simulink model "BD_CONV2"  (Simulink 4.1.1)
settings: Solver=ode1  SolverMode=SingleTasking  StartTime=0.0  StopTime=max(cyc_mph(:,1))  FixedStep=1  MaxStep=1  RelTol=1e-3  AbsTol=1e-3
undefined symbols (not defined in the file): cyc_mph, ess_on, ex_calc, fc_ct_trq, fc_emis, fc_inertia, fc_map_spd, fc_max_trq, fc_spd_scale, fc_trq_scale, fd_inertia, fd_loss, fd_ratio, gb_dnshift_load, gb_dnshift_spd, gb_gears_num, gb_inertia, gb_num_init, gb_ratio, gb_shift_delay, gb_spd_scale, gb_trq_scale, gb_upshift_load, gb_upshift_spd, logFlag, tx_eff_map, tx_map_spd, tx_map_trq, vc_clutch_bool, vc_idle_bool, vc_idle_spd, vc_key_on, vc_launch_spd, veh_air_density, veh_CD, veh_FA, veh_gravity, veh_mass, wh_axle_loss_mass, wh_axle_loss_trq, wh_front_active_bool, wh_inertia, wh_max_front_brake_force, wh_max_rear_brake_force, wh_radius, wh_rear_active_bool, wh_slip, wh_slip_force_coeff
libraries: lib_wheel2 x12, lib_drive_cycle2 x2, lib_accessory2 x2, lib_etc x2, lib_interactive x1, lib_exhaust x1, lib_fuel_converter3 x1, lib_help x1
(part 8 of 11)

== system BD_CONV2/<cs> control strategy/Clutch Control/Clutch Control/clutch control ==
  shifting : Inport  Port=1  LatchInput=off
  gb_trq_in_r : Inport  Port=2  LatchInput=off
  gb_spd_in_r : Inport  Port=3  LatchInput=off
  Block NOTES : Subsystem
      settings: RTWFcnNameOpts=Auto  RTWFileNameOpts=Auto
      mask Display: disp('Block\nNOTES')
  Constant : Constant  Value=1e-3
  Constant1 : Constant  Value=vc_clutch_bool
  Constant2 : Constant  Value=vc_idle_spd
  Constant3 : Constant  Value=1e-3
  Constant4 : Constant  Value=vc_launch_spd
  Constant5 : Constant  Orientation=left  Value=2.5
  Fcn: 1 if clutch disengaged 2 if clutch slipping 3 if clutch engaged : Fcn  Expr=u[1]+2*u[2]*(1-u[1])*(1-u[3])+3*u[3]*(1-u[1])
  Logical Operator : Logic  Operator=AND  Inputs=2
  Logical Operator1 : Logic  Operator=OR  Inputs=2
  Memory : Memory  Orientation=left  X0=1+(2*(cyc_mph(1,2)>0))  InheritSampleTime=off
      settings: RTWStateStorageClass=Auto
  Mux : Mux  Inputs=3
      settings: DisplayOption=none
  Relational Operator : RelationalOperator  Operator=<=
  Relational Operator1 : RelationalOperator  Operator=<
  Relational Operator2 : RelationalOperator  Operator=>
  Relational Operator3 : RelationalOperator  Operator=<
  clutch disengaged : Logic  Operator=OR  Inputs=2
  clutch engaged : Logic  Operator=NOR  Inputs=2
  clutch slipping : Logic  Operator=AND  Inputs=3
  clutch was NOT fully engaged during last time step : RelationalOperator  Orientation=left  Operator=<
  gearbox speed estimator : Subsystem
      settings: RTWFcnNameOpts=Auto  RTWFileNameOpts=Auto
  clutch state : Outport  Port=1
  wires:
  gearbox speed estimator/1(Out1) -> Relational Operator3/1, Relational Operator1/1
  gb_spd_in_r/1 -> gearbox speed estimator/1(gb_spd_in_r if no gear change)
  shifting/1 -> clutch disengaged/1
  Logical Operator/1 -> clutch disengaged/2
  gb_trq_in_r/1 -> Relational Operator2/1, Relational Operator/1
  Logical Operator1/1 -> Logical Operator/2
  Relational Operator/1 -> Logical Operator/1
  Constant/1 -> Relational Operator/2
  Constant1/1 -> Logical Operator1/1
  clutch was NOT fully engaged during last time step/1 -> clutch slipping/3
  Constant5/1 -> clutch was NOT fully engaged during last time step/2
  Memory/1 -> clutch was NOT fully engaged during last time step/1
  Relational Operator3/1 -> clutch slipping/2
  Constant4/1 -> Relational Operator3/2
  clutch slipping/1 -> Mux/2, clutch engaged/2
  Relational Operator2/1 -> clutch slipping/1
  Constant3/1 -> Relational Operator2/2
  Fcn: 1 if clutch disengaged 2 if clutch slipping 3 if clutch engaged/1 -> Memory/1, clutch state/1
  clutch disengaged/1 -> Mux/1, clutch engaged/1
  clutch engaged/1 -> Mux/3
  Mux/1 -> Fcn: 1 if clutch disengaged 2 if clutch slipping 3 if clutch engaged/1
  Constant2/1 -> Relational Operator1/2
  Relational Operator1/1 -> Logical Operator1/2

== system BD_CONV2/<cs> control strategy/Clutch Control/Clutch Control/repeated cycle:  speed required at end of NEXT step ==
  Clock : Clock
      settings: DisplayTime=off  Decimation=10
  Fcn1 : Fcn  Expr=rem(u[1],period)
  Look-Up Table : Lookup  InputValues=t  OutputValues=y
  Memory : Memory  X0=-0.1  InheritSampleTime=off
      settings: RTWStateStorageClass=Auto
  Sum : Sum  Inputs=+-  SaturateOnIntegerOverflow=on
  Sum1 : Sum  Inputs=++  SaturateOnIntegerOverflow=on
  out_1 : Outport  Port=1  InitialOutput=0
  wires:
  Clock/1 -> Sum/1, Memory/1, Fcn1/1
  Memory/1 -> Sum/2
  Sum/1 -> Sum1/2
  Fcn1/1 -> Sum1/1
  Look-Up Table/1 -> out_1/1
  Sum1/1 -> Look-Up Table/1

== system BD_CONV2/<cs> control strategy/Fuel Converter Control conventional ic engine/conventional IC engine/Fuel Converter Control ==
  note: Controls for Fuel Converter
  note: This is just to give a matching FROM block for the sensors
  note: calculated above
  note: calculated above
  clutch_state : Inport  Port=1  LatchInput=off
  mpha(t-1) (prev) : Inport  Port=2  LatchInput=off
  gear_ratio : Inport  Port=3  LatchInput=off
  current_veh_mass : Inport  Port=4  LatchInput=off
  veh_spd_a_rec(t-1) (prev) : Inport  Port=5  LatchInput=off
  cyc_mph_r(t-1) (prev) : Inport  Port=6  LatchInput=off
  acc_mech_trq_est : Inport  Port=7  LatchInput=off
  fcSensors : Inport  Port=8  LatchInput=off
  shifting : Inport  Port=9  LatchInput=off
  v_prev : Inport  Port=10  LatchInput=off
  Constant : Constant  Value=1.1
  Constant1 : Constant  Value=vc_idle_bool
  Logical Operator1 : Logic  Operator=AND  Inputs=2
  Logical Operator2 : Logic  Operator=OR  Inputs=2
  Logical Operator3 : Logic  Operator=OR  Inputs=2
  Logical Operator7 : Logic  Operator=AND  Inputs=2
  Memory : Memory  Orientation=left  X0=0  InheritSampleTime=off
      settings: RTWStateStorageClass=Auto
  Terminator : Terminator
  clutch slipping or engaged : RelationalOperator  Operator=>
  key_on : Subsystem  mask(Repeating table){@1=vc_key_on(:,1), @2=vc_key_on(:,2)}
      mask prompts: @1 "Time values:"; @2 "Output values:"
      mask help:
      | Repeating table.
      | Enter values of time and output for first cycle.
      mask init:
      | period = max(@1); t = @1; y = @2;
      settings: RTWFcnNameOpts=Auto  RTWFileNameOpts=Auto
      mask Help: Repeats cycle given in table. Time values should be monotonically increasing.
  clutch state out : Outport  Port=1
  miles per hour out : Outport  Port=2
  gear_ratio out : Outport  Port=3
  current veh mass out : Outport  Port=4
  veh spd a rec out : Outport  Port=5
  cyc_mph_r out : Outport  Port=6
  acc_mech_trq_est out : Outport  Port=7
  engine_on out : Outport  Port=8
  key_on out : Outport  Port=9
  v_prev out : Outport  Port=10
  wires:
  gear_ratio/1 -> gear_ratio out/1  "gear_ratio"
  [clutch_state] -> clutch slipping or engaged/1
  Constant1/1 -> Logical Operator2/2
  Constant/1 -> clutch slipping or engaged/2
  clutch slipping or engaged/1 -> Logical Operator2/1
  Logical Operator1/1 -> Logical Operator3/1
  Logical Operator2/1 -> Logical Operator1/2
  [shifting] -> Logical Operator7/1
  Memory/1 -> Logical Operator7/2
  Logical Operator7/1 -> Logical Operator3/2
  Logical Operator3/1 -> [engine_on], Memory/1
  key_on/1(out_1) -> Logical Operator1/1, [key_on]
  fcSensors/1 -> Terminator/1
  shifting/1 -> [shifting]
  clutch_state/1 -> [clutch_state]
  mpha(t-1) (prev)/1 -> miles per hour out/1  "mpha_prev"
  current_veh_mass/1 -> current veh mass out/1  "current_veh_mass"
  veh_spd_a_rec(t-1) (prev)/1 -> veh spd a rec out/1  "veh_spd_a_rec_prev"
  cyc_mph_r(t-1) (prev)/1 -> cyc_mph_r out/1  "cyc_mph_r_prev"
  acc_mech_trq_est/1 -> acc_mech_trq_est out/1  "acc_mech_trq_est"
  v_prev/1 -> v_prev out/1  "v_prev"
  [clutch_state] -> clutch state out/1  "clutch_state"
  [engine_on] -> engine_on out/1  "engine_on"
  [key_on] -> key_on out/1  "key_on"

== system BD_CONV2/<cs> control strategy/Gearbox Control manual shift logic/manual shift logic/gearbox  control ==
  note: local GOTO blocks:
  gb_trq_out_r : Inport  Port=1  LatchInput=off
  gb_spd_out_r : Inport  Port=2  LatchInput=off
  prev. Pout/Pin : Inport  Port=3  LatchInput=off
  tires are at traction limit : Inport  Port=4  LatchInput=off
  Block NOTES : Subsystem
      settings: RTWFcnNameOpts=Auto  RTWFileNameOpts=Auto
      mask Display: disp('Block\nNOTES')
  Constant : Constant  Orientation=left  Value=1
  Fcn : Fcn  Expr=1/u
  Fcn1 : Fcn  Orientation=up  Expr=1/u
  Gain1 : Gain  Gain=-1  Multiplication=Element-wise(K.*u)  SaturateOnIntegerOverflow=on
  Product2 : Product  Inputs=*/  Multiplication=Element-wise(.*)  SaturateOnIntegerOverflow=on
  Product3 : Product  Inputs=2  Multiplication=Element-wise(.*)  SaturateOnIntegerOverflow=on
  Rate Limiter : RateLimiter  Orientation=left  RisingSlewLimit=1/(gb_shift_delay+eps)  FallingSlewLimit=-1/(gb_shift_delay+eps)
  Saturation : Saturate  UpperLimit=1  LowerLimit=0.2  LinearizeAsGain=on
  Saturation1 : Saturate  UpperLimit=gb_gears_num  LowerLimit=1  LinearizeAsGain=on
  Switch : Switch  Threshold=eps
  allow downshift? : Subsystem
      settings: RTWFcnNameOpts=Auto  RTWFileNameOpts=Auto
  current gear number : Sum  Inputs=++  SaturateOnIntegerOverflow=on
  delta gear number : Switch  Threshold=eps
  downshift  command : Subsystem
      settings: RTWFcnNameOpts=Auto  RTWFileNameOpts=Auto
  engine torque capability : Lookup  Orientation=left  InputValues=fc_map_spd*fc_spd_scale  OutputValues=fc_max_trq*fc_trq_scale+eps
  est eng trq : Sum  Inputs=++  SaturateOnIntegerOverflow=on
  gb_spd_in_r : Product  Inputs=2  Multiplication=Element-wise(.*)  SaturateOnIntegerOverflow=on
  gear ratio : Lookup  Orientation=left  InputValues=[1:length(gb_ratio)]  OutputValues=gb_ratio
  gear ratio1 : Lookup  InputValues=[1:length(gb_ratio)]  OutputValues=gb_ratio
  gearbox speed estimator : Subsystem
      settings: RTWFcnNameOpts=Auto  RTWFileNameOpts=Auto
  load=T/ (maxT at spd) : Saturate  UpperLimit=1  LowerLimit=0  LinearizeAsGain=on
  prev gear number : Memory  Orientation=left  X0=gb_num_init  InheritSampleTime=off
      settings: RTWStateStorageClass=Auto
  prev gear ratio : Memory  Orientation=left  X0=gb_ratio(gb_num_init)  InheritSampleTime=off
      settings: RTWStateStorageClass=Auto
  shifting1 : Subsystem
      settings: RTWFcnNameOpts=Auto  RTWFileNameOpts=Auto
  upshift  command : Subsystem
      settings: RTWFcnNameOpts=Auto  RTWFileNameOpts=Auto
  ~gb_trq_in_r : Product  Inputs=3  Multiplication=Element-wise(.*)  SaturateOnIntegerOverflow=on
  gear ratio2 : Outport  Port=1  InitialOutput=0
  shifting : Outport  Port=2  InitialOutput=0
  gear number : Outport  Port=3  InitialOutput=0
  wires:
  [acc_mech_trq_est] -> est eng trq/2
  shifting1/1(out_1) -> shifting/1
  gear ratio1/1 -> gear ratio2/1
  current gear number/1 -> Saturation1/1
  Saturation/1 -> Fcn/1
  prev. Pout/Pin/1 -> Saturation/1
  gb_trq_out_r/1 -> ~gb_trq_in_r/1
  upshift  command/1(command) -> delta gear number/1, delta gear number/2
  downshift  command/1(command) -> Gain1/1
  Fcn1/1 -> ~gb_trq_in_r/3
  engine torque capability/1 -> Product2/2
  Fcn/1 -> ~gb_trq_in_r/2
  Saturation1/1 -> prev gear number/1, gear ratio1/1, gear number/1, Rate Limiter/1, shifting1/1(gear number)
  prev gear number/1 -> allow downshift?/1(prev gearnum), upshift  command/1(prev gear number), downshift  command/1(prev gear number), current gear number/1
  Product2/1 -> load=T/ (maxT at spd)/1
  Constant/1 -> Switch/1
  tires are at traction limit/1 -> Switch/2
  Rate Limiter/1 -> gear ratio/1
  gb_spd_out_r/1 -> gb_spd_in_r/1
  gb_spd_in_r/1 -> gearbox speed estimator/1(gb_spd_in_r if no gear change)
  gear ratio/1 -> prev gear ratio/1
  prev gear ratio/1 -> gb_spd_in_r/2, Fcn1/1
  Gain1/1 -> Product3/2
  Product3/1 -> delta gear number/3
  allow downshift?/1(allow shift) -> Product3/1
  gearbox speed estimator/1(Out1) -> engine torque capability/1, downshift  command/3(engine speed), upshift  command/3(engine speed)
  ~gb_trq_in_r/1 -> est eng trq/1
  est eng trq/1 -> Product2/1
  load=T/ (maxT at spd)/1 -> Switch/3
  Switch/1 -> upshift  command/2(engine load), downshift  command/2(engine load)
  delta gear number/1 -> current gear number/2

== system BD_CONV2/ACC MECH <accm>/mechanical accessory model and interface/Mechanical Accessory model/Block NOTES ==
  note: In this model, only one speed is used to predict accessory
      | loading. The forward model is "dummied" out.
  note: A third input is given for accessory load speed. This is done so that
      | the accessory block can use fc_spd_est which is an estimated vehicle speed
      | (equal to fc_spd_out under normal circumstances).
      | Using fc_spd_est provides total compatibility with ADVISOR v3.2
  note: In terms of an interface, the model assumes belt-driven mechanical loads
      | that run off of a prime mover shaft (e.g., engine shaft)
      |
      | This model takes in requested driveline torque and speed requests and
      | augments torque due to belt driven accessories.
      |
      | The torque passed along down to the driveline is only torque to move the
      | vehicle.
  note: This is the mechanical auxiliary loads model.

== system BD_CONV2/ACC MECH <accm>/mechanical accessory model and interface/Mechanical Accessory model/backward model ==
  note: Power, W, input to accessory
  note: T, Nm, shaft out
  note: T, Nm, driveline
  note: T, Nm, accessory
  note: w_apu, rad/s
  trq1 : Inport  Port=1  LatchInput=off
  spd_in : Inport  Port=2  LatchInput=off
  Product : Product  Inputs=**  Multiplication=Element-wise(.*)  SaturateOnIntegerOverflow=on
  Product1 : Product  Inputs=**  Multiplication=Element-wise(.*)  SaturateOnIntegerOverflow=on
  Sum : Sum  Inputs=|++  SaturateOnIntegerOverflow=on
  enhancedToWorkspace : Subsystem  TreatAsAtomicUnit=on  mask(enhancedToWorkspace){generalName=generalName, specificName=mech_pwr_r, logFlag=logFlag}
      mask prompts: generalName "General Name [char-evaluated]"; specificName "Specific Name [char-literal]"; logFlag "Enable flag (1=on,0=off)"
      mask help: A wrapper for the Simulink "To Workspace" block that allows you to evaluate the name of the variable to log to workspace. This is useful to avoid the double logging errors that occur when you pull in two library models that attempt to log to the same variable.
      mask init:
      | enhancedToWsMaker
      settings: CopyFcn=breakLinkCopyFcn  ParentCloseFcn=breakLinkParCloseFcn  RTWFcnNameOpts=Auto  RTWFileNameOpts=Auto
      mask Help:
      | <h2>Enhanced To Workspace Block</h2>
      | <h3>Parameters</h3>
      | <UL>
      | <li><b>General Name:</b> This is the more general name of the variable. Variables are saved to the workspace as <i>generalName_specificName</i>. Note that this is an evaluated variable. If you would like to type in the value directly, it must be surrounded with single quotes. Otherwise you can input the name of a variable containing a char string.</li>
      | <li><b>Specific Name:</b> This is the specific name of the variable. Note that this is input as a char literal (i.e., you don't need quotes).</li>
      | <li><b>Enable Flag:</b> This flag should have the value of 0 or 1. If 0, the variable will not be logged to the workspace. If 1, the variable will be logged. This is done so that variable logging can be turned off to improve speed.</li>
      | </ul>
      | <h3>Overview</h3>
      | <p>The enhanced to workspace block was put together to allow one to dynamically resolve variable names at run time in simulink. This is most powerful when used in conjunction with a masked subsystem to allow multiple instances of that masked subsytem to be used in the same model. The strategy is to set the generalName in the block mask which will allow the block to change the general name for all variable logging on the fly.
      | <h3>Helper Files</h3>
      | <p>Three m-files are required by the enhancedToWorkspace block. These files are located in the &lt; ADVISOR root &gt;/GUI directory :
      | <ul>
      | <li><i>enhancedToWsMaker.m</i> This file runs the mask initialization for the block</li>
      | <li><i>breakLinkCopyFcn.m</i> This file is used by the block callback when the simulink block is copied. It is necessary to break the link to the enhancedToWorkspace similar to the To Workspace block in order for it to be able to configure itself. (Try copying simulink's To Workspace block--it is impossible to make a link)</li>
      | <li><i>breakLinkParCloseFcn.m</i> This file is similar to the breakLinkCopyFcn and is used when a parent system is closed</li>
      | </ul>
      | <hr>
      | 
      | <p>Created 2003-Jan-21, Michael Patrick O'Keefe, NREL</p>
      | 
      | <!--
      | <VARDEF>
      | <H3>var_name</H3>
      | <UL>
      | <LI><B>data type</B> data type here</LI>
      | <LI><B>units</B> units here</LI>
      | <LI><B>vehicle type</B> vehicle type here</LI>
      | <LI><B>description</B> description here</LI>
      | </UL>
      | </VARDEF>
      | -->
      mask Display: disp([generalName,'_',specificName])
  enhancedToWorkspace1 : Subsystem  TreatAsAtomicUnit=on  mask(enhancedToWorkspace){generalName=generalName, specificName=mech_trq_r, logFlag=logFlag}
      mask prompts: generalName "General Name [char-evaluated]"; specificName "Specific Name [char-literal]"; logFlag "Enable flag (1=on,0=off)"
      mask help: A wrapper for the Simulink "To Workspace" block that allows you to evaluate the name of the variable to log to workspace. This is useful to avoid the double logging errors that occur when you pull in two library models that attempt to log to the same variable.
      mask init:
      | enhancedToWsMaker
      settings: CopyFcn=breakLinkCopyFcn  ParentCloseFcn=breakLinkParCloseFcn  RTWFcnNameOpts=Auto  RTWFileNameOpts=Auto
      mask Help:
      | <h2>Enhanced To Workspace Block</h2>
      | <h3>Parameters</h3>
      | <UL>
      | <li><b>General Name:</b> This is the more general name of the variable. Variables are saved to the workspace as <i>generalName_specificName</i>. Note that this is an evaluated variable. If you would like to type in the value directly, it must be surrounded with single quotes. Otherwise you can input the name of a variable containing a char string.</li>
      | <li><b>Specific Name:</b> This is the specific name of the variable. Note that this is input as a char literal (i.e., you don't need quotes).</li>
      | <li><b>Enable Flag:</b> This flag should have the value of 0 or 1. If 0, the variable will not be logged to the workspace. If 1, the variable will be logged. This is done so that variable logging can be turned off to improve speed.</li>
      | </ul>
      | <h3>Overview</h3>
      | <p>The enhanced to workspace block was put together to allow one to dynamically resolve variable names at run time in simulink. This is most powerful when used in conjunction with a masked subsystem to allow multiple instances of that masked subsytem to be used in the same model. The strategy is to set the generalName in the block mask which will allow the block to change the general name for all variable logging on the fly.
      | <h3>Helper Files</h3>
      | <p>Three m-files are required by the enhancedToWorkspace block. These files are located in the &lt; ADVISOR root &gt;/GUI directory :
      | <ul>
      | <li><i>enhancedToWsMaker.m</i> This file runs the mask initialization for the block</li>
      | <li><i>breakLinkCopyFcn.m</i> This file is used by the block callback when the simulink block is copied. It is necessary to break the link to the enhancedToWorkspace similar to the To Workspace block in order for it to be able to configure itself. (Try copying simulink's To Workspace block--it is impossible to make a link)</li>
      | <li><i>breakLinkParCloseFcn.m</i> This file is similar to the breakLinkCopyFcn and is used when a parent system is closed</li>
      | </ul>
      | <hr>
      | 
      | <p>Created 2003-Jan-21, Michael Patrick O'Keefe, NREL</p>
      | 
      | <!--
      | <VARDEF>
      | <H3>var_name</H3>
      | <UL>
      | <LI><B>data type</B> data type here</LI>
      | <LI><B>units</B> units here</LI>
      | <LI><B>vehicle type</B> vehicle type here</LI>
      | <LI><B>description</B> description here</LI>
      | </UL>
      | </VARDEF>
      | -->
      mask Display: disp([generalName,'_',specificName])
  mechanical accessories (Nm) : Subsystem  BlockChoice=Mechanical Accessories: Const Mech Var Elect
      settings: AttributesFormatString=%<BlockChoice>  MemberBlocks=Mechanical Accessories: Const Mech Var Elect,Mechanical Accessories: Constant Mechanical & Electrical,Mechanical Accessories: Speed Dependant and Variable Electrical,Saber Dual Voltage Cosim,Saber Single Voltage Cosim,SindaTransAC  RTWFcnNameOpts=Auto  RTWFileNameOpts=Auto
      settings: TemplateBlock=|
      | lib_accessory2/ACC MECH
      | models/mechanical accessories (Nm)
      mask Display: image(imread('bdi_acc_pic_cs.bmp'))
  trq2 : Outport  Port=1
  tag scope: acc_mech_pwr_r=scoped, acc_mech_trq_r=scoped
  wires:
  [acc_on] -> Product1/2
  [acc_on] -> Product/1
  mechanical accessories (Nm)/2(P_mech_acc) -> Product1/1
  Product1/1 -> enhancedToWorkspace/1(In1), [acc_mech_pwr_r]
  mechanical accessories (Nm)/1(T_acc) -> Product/2
  Product/1 -> enhancedToWorkspace1/1(In1), [acc_mech_trq_r], Sum/2
  Sum/1 -> trq2/1
  trq1/1 -> Sum/1
  spd_in/1 -> mechanical accessories (Nm)/1(w_APU)

== system BD_CONV2/ACC MECH <accm>/mechanical accessory model and interface/Mechanical Accessory model/f1 ==
  In1 : Inport  Port=1  LatchInput=off
  To Workspace : ToWorkspace  VariableName=acc_mech_pwr_a  SampleTime=-1  SaveFormat=Array
  wires:
  In1/1 -> To Workspace/1

== system BD_CONV2/ACC MECH <accm>/mechanical accessory model and interface/Mechanical Accessory model/f2 ==
  In1 : Inport  Port=1  LatchInput=off
  To Workspace : ToWorkspace  VariableName=acc_mech_trq_a  SampleTime=-1  SaveFormat=Array
  wires:
  In1/1 -> To Workspace/1

== system BD_CONV2/ACC MECH <accm>/mechanical accessory model and interface/Mechanical Accessory model/forward model ==
  note: pm trq a ==> prime mover (engine/fuel converter/input shaft driving accessories) torque achieved
      | acc spd ==> accessory reference shaft speed (may or may not be the same as the engine shaft speed
      | acc trq requested ==> accessory torque requested
  note: acc torque, Nm
  note: NOTES
  note: This simplistic model may not correctly account for accessory torque and/or power
      | when the upstream torque provider is torque or speed limited
  note: Power, W, input to accessory
  note: T, Nm, shaft out
  note: driveline and
      | acc torque, Nm
  note: T, Nm, accessory
  note: acc speed, rad/s
  trq_in : Inport  Port=1  LatchInput=off
  spd_in : Inport  Port=2  LatchInput=off
  acc_trq_req : Inport  Port=3  LatchInput=off
  Product1 : Product  Inputs=**  Multiplication=Element-wise(.*)  SaturateOnIntegerOverflow=on
  Sum : Sum  Inputs=|+-  SaturateOnIntegerOverflow=on
  trq_out : Outport  Port=1
  acc_mech_trq_a : Outport  Port=2
  acc_mech_pwr_a : Outport  Port=3
  wires:
  [pm_trq_a] -> Sum/1
  acc_trq_req/1 -> [acc_trq_r]
  trq_in/1 -> [pm_trq_a]
  [acc_spd] -> Product1/2
  [acc_trq_r] -> Product1/1, Sum/2, acc_mech_trq_a/1
  Product1/1 -> acc_mech_pwr_a/1
  Sum/1 -> trq_out/1
  spd_in/1 -> [acc_spd]

== system BD_CONV2/ACC MECH <accm>/mechanical accessory model and interface/signal annotator/enhancedToWorkspace ==
  In1 : Inport  Port=1  LatchInput=off
  To Workspace : ToWorkspace  VariableName=acc_pre_acc_spd_out_r  SampleTime=-1  SaveFormat=Array
  wires:
  In1/1 -> To Workspace/1

== system BD_CONV2/ACC MECH <accm>/mechanical accessory model and interface/signal annotator/enhancedToWorkspace1 ==
  In1 : Inport  Port=1  LatchInput=off
  To Workspace : ToWorkspace  VariableName=acc_pre_acc_trq_out_r  SampleTime=-1  SaveFormat=Array
  wires:
  In1/1 -> To Workspace/1

== system BD_CONV2/clutch <cl>/clutch model and interface/clutch model/Adjust for Possible Launch Speed Request ==
  note: If the clutch is disengaged, under certain
      | circumstances, we will want to request that
      | the input speed to the clutch be ramped up to a
      | given launch speed (decided by the controller)
      | so that the clutch can subsequently slip and
      | engage with a more realistic speed matching
  Input Speed Request : Inport  Port=1  LatchInput=off
  Constant6 : Constant  Value=1
  Logical Operator : Logic  Operator=AND  Inputs=2
  Switch4 : Switch  Threshold=0.5
  clutch disengaged : RelationalOperator  Operator===
  Input Speed Request Adjusted for Launch Speed : Outport  Port=1
  wires:
  Logical Operator/1 -> Switch4/2
  clutch disengaged/1 -> Logical Operator/2
  [launch_flag] -> Logical Operator/1
  Constant6/1 -> clutch disengaged/2
  [clutch_state] -> clutch disengaged/1
  Input Speed Request/1 -> Switch4/3
  Switch4/1 -> Input Speed Request Adjusted for Launch Speed/1
  [launch_speed] -> Switch4/1

== system BD_CONV2/clutch <cl>/clutch model and interface/clutch model/enhancedToWorkspace ==
  In1 : Inport  Port=1  LatchInput=off
  To Workspace : ToWorkspace  VariableName=cl_pwr_out_a  SampleTime=-1  SaveFormat=Array
  wires:
  In1/1 -> To Workspace/1

== system BD_CONV2/clutch <cl>/clutch model and interface/clutch model/enhancedToWorkspace1 ==
  In1 : Inport  Port=1  LatchInput=off
  To Workspace : ToWorkspace  VariableName=cl_pwr_in_a  SampleTime=-1  SaveFormat=Array
  wires:
  In1/1 -> To Workspace/1

== system BD_CONV2/clutch <cl>/clutch model and interface/clutch model/enhancedToWorkspace2 ==
  In1 : Inport  Port=1  LatchInput=off
  To Workspace : ToWorkspace  VariableName=cl_trq_out_r  SampleTime=-1  SaveFormat=Array
  wires:
  In1/1 -> To Workspace/1

== system BD_CONV2/clutch <cl>/clutch model and interface/clutch model/enhancedToWorkspace3 ==
  In1 : Inport  Port=1  LatchInput=off
  To Workspace : ToWorkspace  VariableName=cl_spd_out_r  SampleTime=-1  SaveFormat=Array
  wires:
  In1/1 -> To Workspace/1

== system BD_CONV2/clutch <cl>/clutch model and interface/clutch model/enhancedToWorkspace4 ==
  In1 : Inport  Port=1  LatchInput=off
  To Workspace : ToWorkspace  VariableName=cl_spd_in_r  SampleTime=-1  SaveFormat=Array
  wires:
  In1/1 -> To Workspace/1

== system BD_CONV2/clutch <cl>/clutch model and interface/clutch model/enhancedToWorkspace5 ==
  In1 : Inport  Port=1  LatchInput=off
  To Workspace : ToWorkspace  VariableName=cl_trq_in_r  SampleTime=-1  SaveFormat=Array
  wires:
  In1/1 -> To Workspace/1

== system BD_CONV2/clutch <cl>/clutch model and interface/clutch model/enhancedToWorkspace6 ==
  In1 : Inport  Port=1  LatchInput=off
  To Workspace : ToWorkspace  VariableName=cl_trq_out_a  SampleTime=-1  SaveFormat=Array
  wires:
  In1/1 -> To Workspace/1

== system BD_CONV2/clutch <cl>/clutch model and interface/clutch model/enhancedToWorkspace7 ==
  In1 : Inport  Port=1  LatchInput=off
  To Workspace : ToWorkspace  VariableName=cl_spd_out_a  SampleTime=-1  SaveFormat=Array
  wires:
  In1/1 -> To Workspace/1

== system BD_CONV2/clutch <cl>/clutch model and interface/clutch model/enhancedToWorkspace8 ==
  In1 : Inport  Port=1  LatchInput=off
  To Workspace : ToWorkspace  VariableName=cl_spd_in_a  SampleTime=-1  SaveFormat=Array
  wires:
  In1/1 -> To Workspace/1

== system BD_CONV2/clutch <cl>/clutch model and interface/clutch model/enhancedToWorkspace9 ==
  In1 : Inport  Port=1  LatchInput=off
  To Workspace : ToWorkspace  VariableName=cl_trq_in_a  SampleTime=-1  SaveFormat=Array
  wires:
  In1/1 -> To Workspace/1

== system BD_CONV2/clutch <cl>/clutch model and interface/clutch model/help ==

== system BD_CONV2/final drive <fd>/final drive model & interface/final drive model/Block NOTES ==
  note: The inertia torque is the input torque required to accelerate the
      | final drive's inertia as measured on the input side.
  note: The loss torque is zero when the gears are not turning,
      | and is applied at the input side of the gear reduction.
  note: This final drive model includes loss data, rotational inertia, and a gear reduction.

== system BD_CONV2/final drive <fd>/final drive model & interface/final drive model/effect of inertia (Nm) ==
  note: The inertia torque is the input torque required to accelerate the
      | final drive's inertia as measured on the input side.
  fd input speed (rad/s) : Inport  Port=1  LatchInput=off
  Gain : Gain  Gain=fd_inertia  Multiplication=Element-wise(K.*u)  SaturateOnIntegerOverflow=on
  d/dt : Derivative
  drag torque (Nm) : Outport  Port=1  InitialOutput=0
  wires:
  fd input speed (rad/s)/1 -> d/dt/1
  d/dt/1 -> Gain/1
  Gain/1 -> drag torque (Nm)/1

== system BD_CONV2/final drive <fd>/final drive model & interface/final drive model/enhancedToWorkspace ==
  In1 : Inport  Port=1  LatchInput=off
  To Workspace : ToWorkspace  VariableName=fd_trq_in_a  SampleTime=-1  SaveFormat=Array
  wires:
  In1/1 -> To Workspace/1

== system BD_CONV2/final drive <fd>/final drive model & interface/final drive model/enhancedToWorkspace1 ==
  In1 : Inport  Port=1  LatchInput=off
  To Workspace : ToWorkspace  VariableName=fd_spd_in_a  SampleTime=-1  SaveFormat=Array
  wires:
  In1/1 -> To Workspace/1

== system BD_CONV2/final drive <fd>/final drive model & interface/final drive model/enhancedToWorkspace2 ==
  In1 : Inport  Port=1  LatchInput=off
  To Workspace : ToWorkspace  VariableName=fd_spd_out_a  SampleTime=-1  SaveFormat=Array
  wires:
  In1/1 -> To Workspace/1

== system BD_CONV2/final drive <fd>/final drive model & interface/final drive model/enhancedToWorkspace3 ==
  In1 : Inport  Port=1  LatchInput=off
  To Workspace : ToWorkspace  VariableName=fd_trq_out_a  SampleTime=-1  SaveFormat=Array
  wires:
  In1/1 -> To Workspace/1

== system BD_CONV2/final drive <fd>/final drive model & interface/final drive model/enhancedToWorkspace4 ==
  In1 : Inport  Port=1  LatchInput=off
  To Workspace : ToWorkspace  VariableName=fd_spd_in_r  SampleTime=-1  SaveFormat=Array
  wires:
  In1/1 -> To Workspace/1

== system BD_CONV2/final drive <fd>/final drive model & interface/final drive model/enhancedToWorkspace5 ==
  In1 : Inport  Port=1  LatchInput=off
  To Workspace : ToWorkspace  VariableName=fd_trq_in_r  SampleTime=-1  SaveFormat=Array
  wires:
  In1/1 -> To Workspace/1

== system BD_CONV2/final drive <fd>/final drive model & interface/final drive model/enhancedToWorkspace6 ==
  In1 : Inport  Port=1  LatchInput=off
  To Workspace : ToWorkspace  VariableName=fd_trq_out_r  SampleTime=-1  SaveFormat=Array
  wires:
  In1/1 -> To Workspace/1

== system BD_CONV2/final drive <fd>/final drive model & interface/final drive model/enhancedToWorkspace7 ==
  In1 : Inport  Port=1  LatchInput=off
  To Workspace : ToWorkspace  VariableName=fd_spd_out_r  SampleTime=-1  SaveFormat=Array
  wires:
  In1/1 -> To Workspace/1

== system BD_CONV2/final drive <fd>/final drive model & interface/final drive model/help ==

== system BD_CONV2/final drive <fd>/final drive model & interface/final drive model/loss (Nm) ==
  note: The loss torque is zero when the gears are not turning,
      | and is applied at the input side of the gear reduction.
  fd output speed (rad/s) : Inport  Port=1  LatchInput=off
  Constant : Constant  Orientation=up  Value=0
  Switch : Switch  Threshold=eps
  final drive loss torque (Nm) : Constant  Value=fd_loss
  drag torque (Nm) : Outport  Port=1  InitialOutput=0
  wires:
  Constant/1 -> Switch/3
  fd output speed (rad/s)/1 -> Switch/2
  Switch/1 -> drag torque (Nm)/1
  final drive loss torque (Nm)/1 -> Switch/1

== system BD_CONV2/fuel converter <fc>/IC Engine Model  &  Interface/ic engine model/Block NOTES ==
  note: This block models the internal combustion engine, and includes inertia effects,
      | performance limits, accessory loads, and temperature transient effects on fuel
      | use, engine-out emissions, and catalyst efficiency.  There are 'leads' to the
      | engine controller here, which controller determines whether the engine is on.

== system BD_CONV2/fuel converter <fc>/IC Engine Model  &  Interface/ic engine model/Speed Limits ==
  Speed Requested : Inport  Port=1  LatchInput=off
  Constant : Constant  Value=0
  Speed Limits : Saturate  UpperLimit=max(fc_map_spd)*fc_spd_scale  LowerLimit=vc_idle_spd*vc_idle_bool  LinearizeAsGain=on
  "if engine is not on, speed is zero" : Switch  Threshold=0.5
  Limited Speed Request : Outport  Port=1
  wires:
  Constant/1 -> "if engine is not on, speed is zero"/3
  [engine_on] -> "if engine is not on, speed is zero"/2
  "if engine is not on, speed is zero"/1 -> Limited Speed Request/1
  Speed Limits/1 -> "if engine is not on, speed is zero"/1
  Speed Requested/1 -> Speed Limits/1

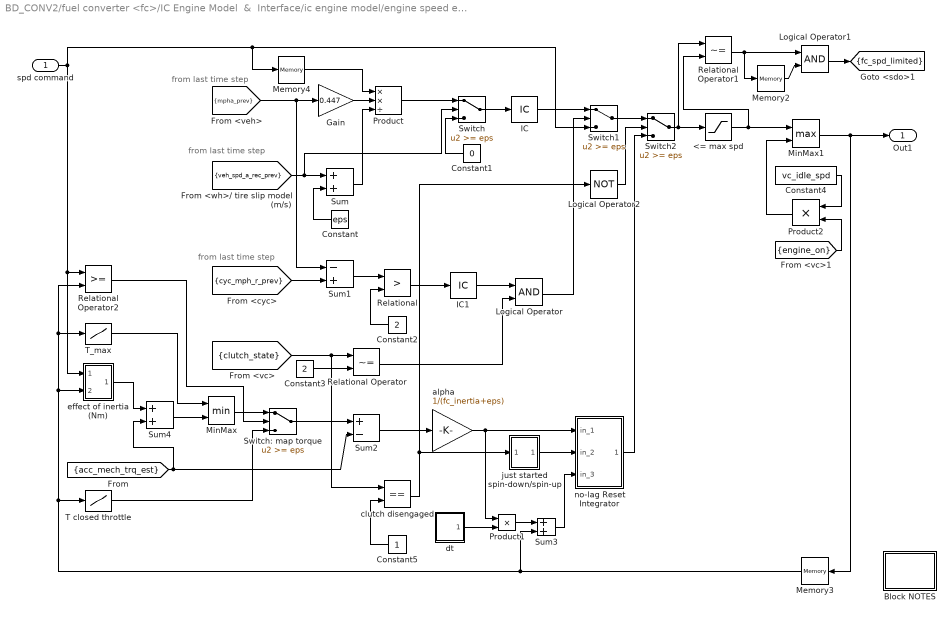
== system BD_CONV2/fuel converter <fc>/IC Engine Model  &  Interface/ic engine model/engine speed estimator ==
  note: from last time step
  note: from last time step
  note: from last time step
  spd command : Inport  Port=1  LatchInput=off
  <= max spd : Saturate  UpperLimit=max(fc_map_spd)*fc_spd_scale  LowerLimit=-inf  LinearizeAsGain=on
  Block NOTES : Subsystem
      settings: RTWFcnNameOpts=Auto  RTWFileNameOpts=Auto
      mask Display: disp('Block\nNOTES')
  Constant : Constant  Orientation=left  Value=eps
  Constant1 : Constant  Orientation=left  Value=0
  Constant2 : Constant  Orientation=left  Value=2
  Constant3 : Constant  Value=2
  Constant4 : Constant  Value=vc_idle_spd
  Constant5 : Constant  Orientation=left  Value=1
  Gain : Gain  Gain=0.447  Multiplication=Element-wise(K.*u)  SaturateOnIntegerOverflow=on
  IC : InitialCondition  Value=cyc_mph(1,2)*0.447/wh_radius*fd_ratio*gb_ratio(gb_num_init)
  IC1 : InitialCondition  Value=0
  Logical Operator : Logic  Operator=AND  Inputs=2
  Logical Operator1 : Logic  Operator=AND  Inputs=2
  Logical Operator2 : Logic  Operator=NOT  Inputs=1
  Memory2 : Memory  X0=0  InheritSampleTime=off
      settings: RTWStateStorageClass=Auto
  Memory3 : Memory  Orientation=left  X0=cyc_mph(1,2)*0.447/wh_radius*fd_ratio*max(gb_ratio)  InheritSampleTime=off
      settings: RTWStateStorageClass=Auto
  Memory4 : Memory  X0=0  InheritSampleTime=off
      settings: RTWStateStorageClass=Auto
  MinMax : MinMax  Function=min  Inputs=2
  MinMax1 : MinMax  Function=max  Inputs=2
  Product : Product  Inputs=**/  Multiplication=Element-wise(.*)  SaturateOnIntegerOverflow=on
  Product1 : Product  Inputs=2  Multiplication=Element-wise(.*)  SaturateOnIntegerOverflow=on
  Product2 : Product  Orientation=left  Inputs=2  Multiplication=Element-wise(.*)  SaturateOnIntegerOverflow=on
  Relational : RelationalOperator  Operator=>
  Relational Operator : RelationalOperator  Operator=~=
  Relational Operator1 : RelationalOperator  Operator=~=
  Relational Operator2 : RelationalOperator  Operator=>=
  Sum : Sum  Inputs=++  SaturateOnIntegerOverflow=on
  Sum1 : Sum  Inputs=-+  SaturateOnIntegerOverflow=on
  Sum2 : Sum  Inputs=+-  SaturateOnIntegerOverflow=on
  Sum3 : Sum  Inputs=++  SaturateOnIntegerOverflow=on
  Sum4 : Sum  Inputs=++  SaturateOnIntegerOverflow=on
  Switch : Switch  Threshold=eps
  Switch1 : Switch  Threshold=eps
  Switch2 : Switch  Threshold=eps
  Switch: map torque : Switch  Threshold=eps
  T closed throttle : Lookup  InputValues=fc_map_spd*fc_spd_scale  OutputValues=fc_ct_trq*fc_trq_scale
  T_max : Lookup  InputValues=fc_map_spd*fc_spd_scale  OutputValues=fc_max_trq*fc_trq_scale
  alpha : Gain  Gain=1/(fc_inertia+eps)  Multiplication=Element-wise(K.*u)  SaturateOnIntegerOverflow=on
  clutch disengaged : RelationalOperator  Operator===
  dt : Subsystem
      settings: RTWFcnNameOpts=Auto  RTWFileNameOpts=Auto
  effect of inertia (Nm) : Subsystem
      settings: RTWFcnNameOpts=Auto  RTWFileNameOpts=Auto
  just started spin-down/spin-up : Subsystem
      settings: RTWFcnNameOpts=Auto  RTWFileNameOpts=Auto
  no-lag Reset Integrator : Subsystem  mask(No-lag Reset Integrator){@1=vc_idle_spd}
      mask prompts: @1 "Initial Value"
      mask help: No-lag Reset Integrator
      mask init:
      | initval=@1;
      settings: RTWFcnNameOpts=Auto  RTWFileNameOpts=Auto
      mask Help: Integrates first input using Euler technique.\nAt the time step that input 2 <> zero,\noutput is reset to input 3.
      mask Display: disp('1/s\nw/ reset\nno lag')
  Out1 : Outport  Port=1
  tag scope: fc_spd_limited=scoped
  wires:
  Sum3/1 -> no-lag Reset Integrator/3(in_3)
  just started spin-down/spin-up/1(trigger) -> no-lag Reset Integrator/2(in_2)
  no-lag Reset Integrator/1(out_1) -> Switch2/3
  Logical Operator/1 -> Switch1/2
  Logical Operator2/1 -> Switch2/2
  spd command/1 -> effect of inertia (Nm)/1(req'd spd (rad/s)), Relational Operator2/1, Switch1/3, Memory4/1
  effect of inertia (Nm)/1((Nm)) -> Sum4/1
  Sum4/1 -> MinMax/2
  T_max/1 -> MinMax/1
  MinMax/1 -> Switch: map torque/1
  T closed throttle/1 -> Switch: map torque/3
  Relational Operator2/1 -> Switch: map torque/2
  Switch: map torque/1 -> Sum2/1
  Relational Operator1/1 -> Memory2/1, Logical Operator1/1
  Logical Operator1/1 -> [fc_spd_limited]
  Memory2/1 -> Logical Operator1/2
  Switch2/1 -> Relational Operator1/1, <= max spd/1
  Product2/1 -> MinMax1/2
  MinMax1/1 -> Memory3/1, Out1/1
  Constant4/1 -> Product2/1
  [engine_on] -> Product2/2
  <= max spd/1 -> MinMax1/1, Relational Operator1/2
  Memory3/1 -> T closed throttle/1, effect of inertia (Nm)/2(prev spd), T_max/1, Relational Operator2/2, Sum3/2
  [clutch_state] -> clutch disengaged/1, Relational Operator/1
  clutch disengaged/1 -> just started spin-down/spin-up/1(state), Logical Operator2/1
  Switch1/1 -> Switch2/1
  Constant5/1 -> clutch disengaged/2
  alpha/1 -> no-lag Reset Integrator/1(in_1), Product1/1
  Product1/1 -> Sum3/1
  dt/1(out_1) -> Product1/2
  Sum2/1 -> alpha/1
  Constant3/1 -> Relational Operator/2
  Relational Operator/1 -> Logical Operator/2
  Sum/1 -> Product/3
  Gain/1 -> Product/2
  Switch/1 -> IC/1
  Relational/1 -> IC1/1
  Sum1/1 -> Relational/1
  Constant2/1 -> Relational/2
  [mpha_prev] -> Sum1/1, Gain/1
  [cyc_mph_r_prev] -> Sum1/2
  Constant/1 -> Sum/2
  IC/1 -> Switch1/1
  Constant1/1 -> Switch/3
  [veh_spd_a_rec_prev] -> Switch/2, Sum/1
  Product/1 -> Switch/1
  [acc_mech_trq_est] -> Sum4/2, Sum2/2
  Memory4/1 -> Product/1
  IC1/1 -> Logical Operator/1

== system BD_CONV2/fuel converter <fc>/IC Engine Model  &  Interface/ic engine model/engine torque ==
  fc_trq_out_r : Inport  Port=1  LatchInput=off
  spd command : Inport  Port=2  LatchInput=off
  engine spd : Inport  Port=3  LatchInput=off
  Block NOTES : Subsystem
      settings: RTWFcnNameOpts=Auto  RTWFileNameOpts=Auto
      mask Display: disp('Block\nNOTES')
  Constant1 : Constant  Value=0
  Constant3 : Constant  Value=1
  Logical Operator : Logic  Operator=OR  Inputs=2
  MinMax : MinMax  Function=min  Inputs=2
  MinMax1 : MinMax  Function=max  Inputs=2
  Sum : Sum  Inputs=++  SaturateOnIntegerOverflow=on
  Sum1 : Sum  Inputs=+-  SaturateOnIntegerOverflow=on
  Switch : Switch  Threshold=eps
  Switch1 : Switch  Threshold=eps
  T_closed throttle : Subsystem
      settings: RTWFcnNameOpts=Auto  RTWFileNameOpts=Auto
  T_max : Subsystem
      settings: RTWFcnNameOpts=Auto  RTWFileNameOpts=Auto
  clutch not disengaged : RelationalOperator  Operator=~=
  effect of inertia (Nm) : Subsystem
      settings: RTWFcnNameOpts=Auto  RTWFileNameOpts=Auto
  engine commanded not to decelerate : RelationalOperator  Operator=<=
  limited : RelationalOperator  Operator=~=
  map torque (Nm) : Outport  Port=1
  torque to shaft (Nm) : Outport  Port=2
  tag scope: fc_trq_limited=scoped
  wires:
  spd command/1 -> engine commanded not to decelerate/2
  effect of inertia (Nm)/1((Nm)) -> Sum1/2, Sum/2
  fc_trq_out_r/1 -> Sum/1
  engine spd/1 -> effect of inertia (Nm)/1(engine spd (rad/s)), engine commanded not to decelerate/1, T_max/1(w_APU), T_closed throttle/1(w_APU)
  clutch not disengaged/1 -> Logical Operator/2, Switch1/2
  Switch/1 -> limited/1, MinMax/1
  MinMax1/1 -> Sum1/1, map torque (Nm)/1, limited/2
  T_closed throttle/1(T_closed throttle) -> MinMax1/2, Switch/3
  T_max/1(T_max) -> MinMax/2
  MinMax/1 -> MinMax1/1
  limited/1 -> [fc_trq_limited]
  Logical Operator/1 -> Switch/2
  Sum/1 -> Switch/1
  engine commanded not to decelerate/1 -> Logical Operator/1
  Constant3/1 -> clutch not disengaged/2
  [clutch_state] -> clutch not disengaged/1
  Switch1/1 -> torque to shaft (Nm)/1
  Sum1/1 -> Switch1/1
  Constant1/1 -> Switch1/3

== system BD_CONV2/fuel converter <fc>/IC Engine Model  &  Interface/ic engine model/enhancedToWorkspace ==
  In1 : Inport  Port=1  LatchInput=off
  To Workspace : ToWorkspace  VariableName=fc_spd_out_r  SampleTime=-1  SaveFormat=Array
  wires:
  In1/1 -> To Workspace/1

== system BD_CONV2/fuel converter <fc>/IC Engine Model  &  Interface/ic engine model/enhancedToWorkspace1 ==
  In1 : Inport  Port=1  LatchInput=off
  To Workspace : ToWorkspace  VariableName=fc_spd_est  SampleTime=-1  SaveFormat=Array
  wires:
  In1/1 -> To Workspace/1

== system BD_CONV2/fuel converter <fc>/IC Engine Model  &  Interface/ic engine model/enhancedToWorkspace3 ==
  In1 : Inport  Port=1  LatchInput=off
  To Workspace : ToWorkspace  VariableName=fc_fuel  SampleTime=-1  SaveFormat=Array
  wires:
  In1/1 -> To Workspace/1

== system BD_CONV2/fuel converter <fc>/IC Engine Model  &  Interface/ic engine model/enhancedToWorkspace4 ==
  In1 : Inport  Port=1  LatchInput=off
  To Workspace : ToWorkspace  VariableName=fc_spd_out_a  SampleTime=-1  SaveFormat=Array
  wires:
  In1/1 -> To Workspace/1

== system BD_CONV2/fuel converter <fc>/IC Engine Model  &  Interface/ic engine model/enhancedToWorkspace5 ==
  In1 : Inport  Port=1  LatchInput=off
  To Workspace : ToWorkspace  VariableName=fc_trq_out_a  SampleTime=-1  SaveFormat=Array
  wires:
  In1/1 -> To Workspace/1

== system BD_CONV2/fuel converter <fc>/IC Engine Model  &  Interface/ic engine model/enhancedToWorkspace6 ==
  In1 : Inport  Port=1  LatchInput=off
  To Workspace : ToWorkspace  VariableName=fc_trq_out_r  SampleTime=-1  SaveFormat=Array
  wires:
  In1/1 -> To Workspace/1

== system BD_CONV2/fuel converter <fc>/IC Engine Model  &  Interface/ic engine model/enhancedToWorkspace7 ==
  In1 : Inport  Port=1  LatchInput=off
  To Workspace : ToWorkspace  VariableName=fc_brake_trq  SampleTime=-1  SaveFormat=Array
  wires:
  In1/1 -> To Workspace/1

== system BD_CONV2/fuel converter <fc>/IC Engine Model  &  Interface/ic engine model/fuel use and EO emis Configurable Subsystem ==
  T (Nm) : Inport  Port=1  LatchInput=off
  w (rad/s) : Inport  Port=2  LatchInput=off
  fuel use and EO emis : lib_fuel_converter3/configurable subsystems/fuel use and EO emis
      settings: RTWFcnNameOpts=Auto  RTWFileNameOpts=Auto
  cumulative fuel  use (gal) : Outport  Port=1
  "FC ON?, EOem, MFex, Tex, O2ex" : Outport  Port=2
  Vv,Tfc : Outport  Port=3
  wires:
  T (Nm)/1 -> fuel use and EO emis/1
  w (rad/s)/1 -> fuel use and EO emis/2
  fuel use and EO emis/1 -> cumulative fuel  use (gal)/1
  fuel use and EO emis/2 -> "FC ON?, EOem, MFex, Tex, O2ex"/1
  fuel use and EO emis/3 -> Vv,Tfc/1

== system BD_CONV2/fuel converter <fc>/IC Engine Model  &  Interface/ic engine model/help ==

== system BD_CONV2/gearbox <gb> old/gearbox model & interface/gearbox model/Block NOTES ==
  note: This is a good assumption, at least for the VW 4-speed manual transaxle of SAE 820741.
      | In the VW transaxle, efficiency is fairly independent of torque and speed at high torques.
  note: Available output torque is estimated assuming that the gearbox efficiency for theavailable input
      | torque andspeed is the same as the gearbox efficiency for the REQUESTED input torque.
  note: The inertia torque is the input torque required to accelerate the
      | final drive's inertia as measured on the input side.
  note: The loss torque is zero when the gears are not turning,
      | and is applied at the input side of the gear reduction.
  note: This gearbox model includes loss data, rotational inertia, and a gear reduction.

== system BD_CONV2/gearbox <gb> old/gearbox model & interface/gearbox model/Pout/Pin neglecting inertia ==
  note: Pout/Pin, neglecting inertia, is used to estimate the output torque given the
      | input torque in a very simple forward-facing calculation.
  Tin : Inport  Port=1  LatchInput=off
  Tinertia : Inport  Port=2  LatchInput=off
  Tout : Inport  Port=3  LatchInput=off
  gear ratio : Inport  Port=4  LatchInput=off
  Constant1 : Constant  Orientation=up  Value=0
  Pout/Pin (neglecting inertia) : Subsystem
      settings: RTWFcnNameOpts=Auto  RTWFileNameOpts=Auto
      mask Display: disp('/')
  Product : Product  Inputs=2  Multiplication=Element-wise(.*)  SaturateOnIntegerOverflow=on
  Relational Operator : RelationalOperator  Operator=~=
  Saturation : Saturate  UpperLimit=inf  LowerLimit=0  LinearizeAsGain=on
  Switch : Switch  Threshold=eps
  Tin-Tinertia : Sum  Inputs=+-  SaturateOnIntegerOverflow=on
  make division bombproof : Subsystem
      settings: RTWFcnNameOpts=Auto  RTWFileNameOpts=Auto
  Pout/Pin : Outport  Port=1  InitialOutput=0
  wires:
  gear ratio/1 -> Product/1
  Product/1 -> Pout/Pin (neglecting inertia)/2(in_2)
  Tout/1 -> Pout/Pin (neglecting inertia)/1(in_1)
  Tin-Tinertia/1 -> make division bombproof/1(Tin-Tinertia), Relational Operator/1
  Saturation/1 -> Pout/Pin/1
  Switch/1 -> Saturation/1
  Relational Operator/1 -> Switch/2
  Pout/Pin (neglecting inertia)/1(out_1) -> Switch/1
  Tin/1 -> Tin-Tinertia/1
  Tinertia/1 -> Tin-Tinertia/2
  make division bombproof/1(Out1) -> Product/2
  Constant1/1 -> Relational Operator/2, Switch/3

== system BD_CONV2/gearbox <gb> old/gearbox model & interface/gearbox model/effect of inertia (Nm) ==
  note: The inertia torque is the input torque required to accelerate the
      | gearbox's inertia as measured on the input side.
  gb input speed (rad/s) : Inport  Port=1  LatchInput=off
  Gain : Gain  Gain=gb_inertia  Multiplication=Element-wise(K.*u)  SaturateOnIntegerOverflow=on
  d/dt : Derivative
  drag torque (Nm) : Outport  Port=1  InitialOutput=0
  wires:
  gb input speed (rad/s)/1 -> d/dt/1
  d/dt/1 -> Gain/1
  Gain/1 -> drag torque (Nm)/1

== system BD_CONV2/gearbox <gb> old/gearbox model & interface/gearbox model/enhancedToWorkspace ==
  In1 : Inport  Port=1  LatchInput=off
  To Workspace : ToWorkspace  VariableName=gb_spd_in_a  SampleTime=-1  SaveFormat=Array
  wires:
  In1/1 -> To Workspace/1

== system BD_CONV2/gearbox <gb> old/gearbox model & interface/gearbox model/enhancedToWorkspace1 ==
  In1 : Inport  Port=1  LatchInput=off
  To Workspace : ToWorkspace  VariableName=gb_trq_in_a  SampleTime=-1  SaveFormat=Array
  wires:
  In1/1 -> To Workspace/1

== system BD_CONV2/gearbox <gb> old/gearbox model & interface/gearbox model/enhancedToWorkspace2 ==
  In1 : Inport  Port=1  LatchInput=off
  To Workspace : ToWorkspace  VariableName=gb_spd_out_a  SampleTime=-1  SaveFormat=Array
  wires:
  In1/1 -> To Workspace/1

== system BD_CONV2/gearbox <gb> old/gearbox model & interface/gearbox model/enhancedToWorkspace3 ==
  In1 : Inport  Port=1  LatchInput=off
  To Workspace : ToWorkspace  VariableName=gb_trq_out_a  SampleTime=-1  SaveFormat=Array
  wires:
  In1/1 -> To Workspace/1

== system BD_CONV2/gearbox <gb> old/gearbox model & interface/gearbox model/enhancedToWorkspace4 ==
  In1 : Inport  Port=1  LatchInput=off
  To Workspace : ToWorkspace  VariableName=gb_ni_trq_out_a  SampleTime=-1  SaveFormat=Array
  wires:
  In1/1 -> To Workspace/1

== system BD_CONV2/gearbox <gb> old/gearbox model & interface/gearbox model/enhancedToWorkspace5 ==
  In1 : Inport  Port=1  LatchInput=off
  To Workspace : ToWorkspace  VariableName=gb_spd_in_r  SampleTime=-1  SaveFormat=Array
  wires:
  In1/1 -> To Workspace/1

== system BD_CONV2/gearbox <gb> old/gearbox model & interface/gearbox model/enhancedToWorkspace6 ==
  In1 : Inport  Port=1  LatchInput=off
  To Workspace : ToWorkspace  VariableName=gb_trq_in_r  SampleTime=-1  SaveFormat=Array
  wires:
  In1/1 -> To Workspace/1

== system BD_CONV2/gearbox <gb> old/gearbox model & interface/gearbox model/enhancedToWorkspace7 ==
  In1 : Inport  Port=1  LatchInput=off
  To Workspace : ToWorkspace  VariableName=gb_spd_out_r  SampleTime=-1  SaveFormat=Array
  wires:
  In1/1 -> To Workspace/1

== system BD_CONV2/gearbox <gb> old/gearbox model & interface/gearbox model/enhancedToWorkspace8 ==
  In1 : Inport  Port=1  LatchInput=off
  To Workspace : ToWorkspace  VariableName=gb_trq_out_r  SampleTime=-1  SaveFormat=Array
  wires:
  In1/1 -> To Workspace/1

== system BD_CONV2/gearbox <gb> old/gearbox model & interface/gearbox model/enhancedToWorkspace9 ==
  In1 : Inport  Port=1  LatchInput=off
  To Workspace : ToWorkspace  VariableName=gb_gear_number  SampleTime=-1  SaveFormat=Array
  wires:
  In1/1 -> To Workspace/1
